simulink model "version4_dq"  (R2023b)
settings: Solver=VariableStepAuto  StartTime=0.0  StopTime=40  FixedStep=Ts_power  MaxStep=Ts_power  RelTol=1e-3
undefined symbols (not defined in the file): C_dc, c_dc, c_drt, c_f, C_hv_km, C_p_opt, Cagg, Cbase1v, H_gen, H_vsm, H_WTR, Ibase_hv, Ibase_lv, Ibase_mv, k_d_vsm, k_drt, k_p_p_vsm, k_p_q_vsm, K_pitch, ki_q, Kp_cc, kp_dc, kpu, L_comp, L_d, l_f, l_grid, L_hv_km, L_q, l_t_ehvhv, l_t_hvmv, l_t_mvlv, Lagg, lambda_opt, Lbase1v, length_export, omega_nom, omega_WTR_min, omega_WTR_n, omega_WTR_sl, phase_shift_test_state, phase_shifts, pie_export, pitch_max, pitch_min, Pitchanglevector, Powercoefficient, psi_pm, R_a, r_f, r_grid, R_hv_km, r_t_ehvhv, r_t_hvmv, r_t_mvlv, R_WTR, Ragg, rate_max, rate_min, rocof_slope ... (+22)
libraries: slpidlib x6, simulink x2, spsFirstOrderFilterLib x1, spsSampleandHoldLib x1
(part 1 of 3)
settings Model: SimulationMode=accelerator  Creator=Martin Pedersen  LastModifiedBy=Martin Pedersen
settings SolverCC: DecoupledContinuousIntegration=on
settings DataIOCC: InitialState=xu134_wWT  SaveFinalState=on  SaveFormat=Structure  SaveOutput=off  SignalLogging=off  DSMLogging=off  ReturnWorkspaceOutputs=off

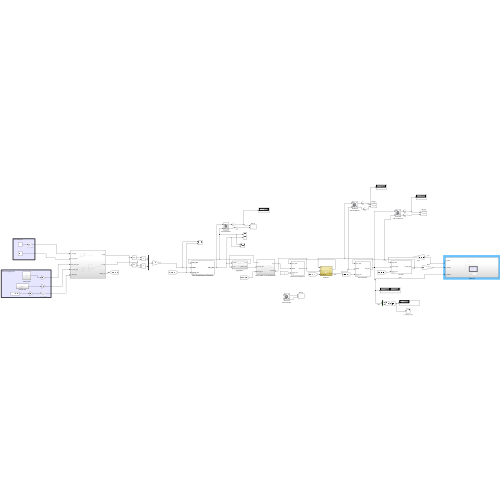
[thumbnail: Simulink's stored preview of the top-level diagram]
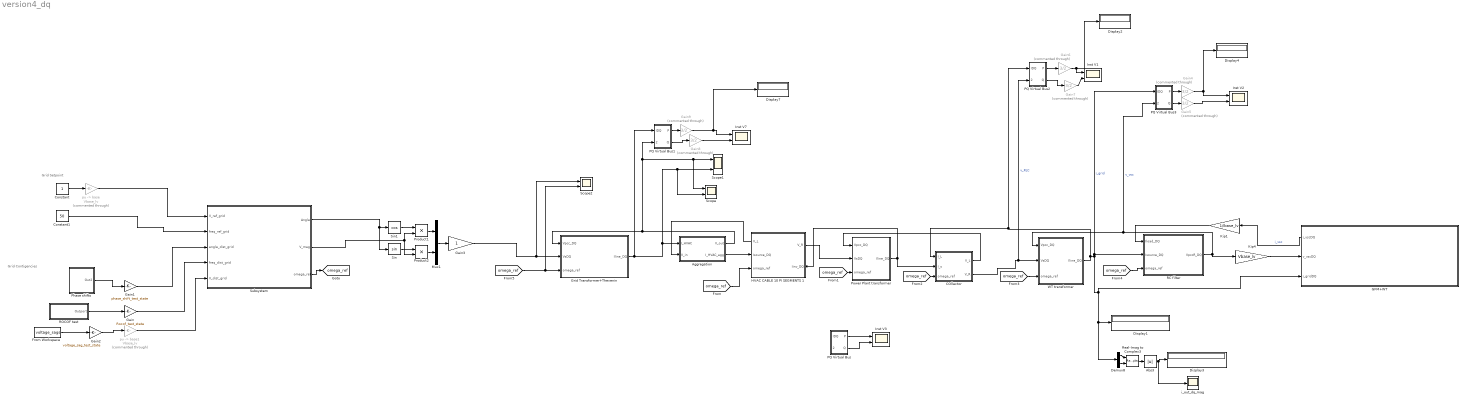
== system version4_dq ==
  note: Grid Contigencies
  note: Grid Setpoint
  Abs3 : Abs
  Aggregation : Subsystem
  COllector : Subsystem
  Constant : Constant
  Constant1 : Constant  Value=50
  Demux8 : Demux  Outputs=[vect vect]
  Display{1..4,7} (5 alike) : Display
  From Workspace : FromWorkspace  VariableName=voltage_sags
  GFM+WT : Subsystem
      settings: PortSchema="{\"entries\":[{\"content\":{\"sides\":[{\"content\":{\"connectorIds\":[\"Out1\",\"In1\",\"In2\"]},\"type\":\"ConnectorPlacement.EquallySpacedRectSide\",\"uuid\":\"bf5f9628-3d85-42f3-b508-ee12217f2900\"},{\"content\":{\"side\":\"RIGHT\"},\"type\":\"ConnectorPlacement.EquallySpacedRectSide\",\"uuid\":\"cb708a52-84f5-4fa8-a61c-6d72c4b87b86\"},{\"content\":{\"side\":\"TOP\"},\"type\":\"ConnectorPlacement.EquallySpacedRectSide\",\"uuid\":\"4c99ef60-a9c3-4166-9091-666343de6d32\"}]},\"type\":\"ConnectorPlacement.EquallySpacedConnector\",\"uuid\":\"b70419d4-69f8-4ca8-a89d-556a2a8c13e9\"}],\"packageUris\":[\"http://schema.mathworks.com/mf0/Connector/R2020b\"],\"version\":\"1.0\"}"
  Gain : Gain  Gain=Rocof_test_state
  Gain1 : Gain  Gain=phase_shift_test_state
  Gain2 : Gain  Gain=voltage_sag_test_state
  Gain3 : Gain  SaturateOnIntegerOverflow=on  OutDataTypeStr=Inherit: Same as input  ParamDataTypeStr=Inherit: Same as input
  Gain{4..9} (6 alike) : Gain  Commented=through  Gain=3/2
  Grid Transformer+Thevenin : Subsystem  mask{Rsource=r_grid+r_t_ehvhv, Lsource=(l_grid+l_t_ehvhv)/omega_nom}
      mask prompts: Rsource "Line resistance"; Lsource "line inductance"
      mask help:
      | RLV_NET is an 3 phase series RL with no virtual resistance termination,
      | 2 voltages as inputs and 1 current output
      mask init:
      | inv_Lsource=1/Lsource;
      mask TypeOptions Rsource: 2/Gain | 3/Gain
      mask TypeOptions Lsource: 7/Gain
  HVAC CABLE 10 PI SEGMENTS 1 : Subsystem
      settings: PortSchema="{\"entries\":[{\"content\":{\"sides\":[{\"content\":{\"connectorIds\":[\"Out2\",\"In1\",\"In2\"]},\"type\":\"ConnectorPlacement.EquallySpacedRectSide\",\"uuid\":\"364e0a5e-18fb-4479-9cea-0c32c2a31756\"},{\"content\":{\"connectorIds\":[\"Out1\",\"In3\"],\"side\":\"RIGHT\"},\"type\":\"ConnectorPlacement.EquallySpacedRectSide\",\"uuid\":\"1b6ff004-fcad-4add-afdc-525ba11bb75d\"},{\"content\":{\"side\":\"TOP\"},\"type\":\"ConnectorPlacement.EquallySpacedRectSide\",\"uuid\":\"fcc13093-d95c-447e-b2c0-1261755b0002\"}]},\"type\":\"ConnectorPlacement.EquallySpacedConnector\",\"uuid\":\"424862c2-d061-479a-b3c0-8c92e3670b7a\"}],\"packageUris\":[\"http://schema.mathworks.com/mf0/Connector/R2020b\"],\"version\":\"1.0\"}"
  Inst V{1..3,7} (4 alike) : Scope  NumInputPorts=2
  Kip1 : Gain  Gain=1/Ibase_lv
  Kip4 : Gain  Gain=Vbase_lv
  Mux1 : Mux  Inputs=2
  PQ Virtual Bus : Subsystem
  PQ Virtual Bus1 : Subsystem
  PQ Virtual Bus2 : Subsystem
  PQ Virtual Bus3 : Subsystem
  Phase shifts : Subsystem
  Power Plant transformer : Subsystem  mask{Rsource=r_t_hvmv, Lsource=l_t_hvmv/omega_nom}
      mask prompts: Rsource "Line resistance"; Lsource "line inductance"
      mask help:
      | RLV_NET is an 3 phase series RL with no virtual resistance termination,
      | 2 voltages as inputs and 1 current output
      mask init:
      | inv_Lsource=1/Lsource;
      mask TypeOptions Rsource: 2/Gain | 3/Gain
      mask TypeOptions Lsource: 7/Gain
  Product1 : Product
  Product2 : Product
  RC filter : Subsystem  mask{Csource=c_f/omega_nom, Rd=0, VD0=1, VQ0=0}
      mask prompts: Csource "Net Capacitance"; Rd "Rdamp"
      mask help:
      | PI network, capacitance to enter is total.
      | Left and right current as input. Left and right voltage as output
      mask init:
      | inv_Csource=1/Csource;
      mask TypeOptions Csource: 8/Gain
      mask TypeOptions Rd: 1/Gain | 2/Gain
      mask TypeOptions VD0: VcpdR_int/InitialCondition
      mask TypeOptions VQ0: VcpqR_int/InitialCondition
  ROCOF test : Subsystem
  Real-Imag to Complex3 : RealImagToComplex
  Scope : Scope  NumInputPorts=2
  Scope1 : Scope  NumInputPorts=2
  Scope2 : Scope  NumInputPorts=2
  Sin : Trigonometry
  Sin1 : Trigonometry  Operator=cos
  Subsystem : Subsystem
  "WT transformer " : Subsystem  mask{Rsource=r_t_mvlv, Lsource=l_t_mvlv/omega_nom}
      mask prompts: Rsource "Line resistance"; Lsource "line inductance"
      mask help:
      | RLV_NET is an 3 phase series RL with no virtual resistance termination,
      | 2 voltages as inputs and 1 current output
      mask init:
      | inv_Lsource=1/Lsource;
      mask TypeOptions Rsource: 2/Gain | 3/Gain
      mask TypeOptions Lsource: 7/Gain
  i_out_dq_mag : Scope
  "pu -> base" : Gain  Commented=through  Gain=Vbase_lv
  "pu -> base1" : Gain  Commented=through  Gain=Vbase_lv
  tag scope: omega_ref=global
  wires:
  Sin/1 -> Product2/1
  Product2/1 -> Mux1/2
  Phase shifts/1(Out2) -> Gain1/1
  Product1/1 -> Mux1/1
  Gain2/1 -> "pu -> base1"/1
  Gain1/1 -> Subsystem/3(angle_dist_grid)
  "pu -> base1"/1 -> Subsystem/5(V_dist_grid)
  ROCOF test/1(Outport) -> Gain/1
  Subsystem/3(omega_ref) -> [omega_ref]
  Subsystem/1(Angle) -> Sin/1, Sin1/1
  Constant/1 -> "pu -> base"/1
  Subsystem/2(V_mag) -> Product2/2, Product1/2
  "pu -> base"/1 -> Subsystem/1(V_ref_grid)
  Mux1/1 -> Gain3/1
  Constant1/1 -> Subsystem/2(freq_ref_grid)
  Sin1/1 -> Product1/1
  Gain/1 -> Subsystem/4(freq_dist_grid)
  From Workspace/1 -> Gain2/1
  Gain3/1 -> Scope2/1, Grid Transformer+Thevenin/2("VsDQ ")
  [omega_ref] -> RC filter/3(omega_ref)
  [omega_ref] -> HVAC CABLE 10 PI SEGMENTS 1/2(omega_ref)
  [omega_ref] -> Power Plant transformer/3(omega_ref)
  PQ Virtual Bus2/2(Q) -> Gain7/1
  PQ Virtual Bus1/1(P) -> Gain9/1
  Gain8/1 -> Inst V7/2
  Gain9/1 -> Display7/1, Inst V7/1
  Real-Imag to Complex3/1 -> Abs3/1
  Gain7/1 -> Inst V1/2
  [omega_ref] -> Scope2/2, Grid Transformer+Thevenin/3(omega_ref)
  COllector/2(V_R) -> PQ Virtual Bus2/2(VDQ), "WT transformer "/2("VsDQ ")  "v_RLC"
  Gain6/1 -> Inst V1/1, Display2/1
  PQ Virtual Bus3/2(Q) -> Gain5/1
  Aggregation/2(I_HVAC_agg) -> HVAC CABLE 10 PI SEGMENTS 1/1("Isource_DQ ")
  PQ Virtual Bus/2(Q) -> Inst V3/2
  PQ Virtual Bus2/1(P) -> Gain6/1
  PQ Virtual Bus3/1(P) -> Gain4/1
  Gain5/1 -> Inst V2/2
  RC filter/1(VpccR_DQ) -> "WT transformer "/1(Vpcc_DQ), PQ Virtual Bus3/2(VDQ), Kip4/1  "v_vsc"
  [omega_ref] -> COllector/3(omega_ref)
  Demux8/2 -> Real-Imag to Complex3/2
  [omega_ref] -> "WT transformer "/3(omega_ref)
  GFM+WT/1(i_vscDQ) -> Kip1/1  "i_vsc"
  HVAC CABLE 10 PI SEGMENTS 1/1(V_R) -> Power Plant transformer/2("VsDQ ")
  Abs3/1 -> i_out_dq_mag/1, Display3/1
  PQ Virtual Bus/1(P) -> Inst V3/1
  Aggregation/1(V_out) -> PQ Virtual Bus1/2(VDQ), Scope/1, Scope1/1, Grid Transformer+Thevenin/1(Vpcc_DQ)
  PQ Virtual Bus1/2(Q) -> Gain8/1
  HVAC CABLE 10 PI SEGMENTS 1/2(V_L) -> Aggregation/2(V_in)
  Demux8/1 -> Real-Imag to Complex3/1
  Gain4/1 -> Display4/1, Inst V2/1
  COllector/1(V_L) -> Power Plant transformer/1(Vpcc_DQ)
  Power Plant transformer/1(Iline_DQ) -> COllector/2(I_s), HVAC CABLE 10 PI SEGMENTS 1/3(Iinv_DQ)
  "WT transformer "/1(Iline_DQ) -> PQ Virtual Bus2/1(IDQ), COllector/1(I_L), GFM+WT/2(i_gridDQ), Demux8/1, Display1/1, RC filter/2("Isource_DQ "), PQ Virtual Bus3/1(IDQ)  "i_grid"
  Grid Transformer+Thevenin/1(Iline_DQ) -> Aggregation/1(I_HVAC), Scope/2, Scope1/2, PQ Virtual Bus1/1(IDQ)
  Kip4/1 -> GFM+WT/1(v_vscDQ)
  Kip1/1 -> RC filter/1(Iload_DQ)

== system version4_dq/Aggregation ==
  I_HVAC : Inport
  V_in : Inport  Port=2
  Demux1 : Demux  Outputs=[vect vect]
  Demux2 : Demux  Outputs=2
  Gain2 : Gain  Gain=1/(1*vect)
  Gain3 : Gain  Gain=ones(vect,1)
  Gain4 : Gain  Gain=ones(vect,1)
  Mux2 : Mux  Inputs=2
  Mux3 : Mux  Inputs=2
  Sum of Elements : Sum  Inputs=+
  Sum of Elements1 : Sum  Inputs=+
  V_out : Outport
  I_HVAC_agg : Outport  Port=2
  wires:
  Mux3/1 -> Gain2/1
  Gain3/1 -> Mux2/1
  Demux2/1 -> Gain3/1
  Sum of Elements1/1 -> Mux3/2
  Gain4/1 -> Mux2/2
  Demux2/2 -> Gain4/1
  Sum of Elements/1 -> Mux3/1
  Gain2/1 -> I_HVAC_agg/1
  V_in/1 -> Demux2/1
  Mux2/1 -> V_out/1
  I_HVAC/1 -> Demux1/1
  Demux1/1 -> Sum of Elements/1
  Demux1/2 -> Sum of Elements1/1

== system version4_dq/COllector ==
  I_L : Inport
  I_s : Inport  Port=2
  omega_ref : Inport  Port=3
  Gain2 : Gain  Gain=1/Vbase_mv
  Gain3 : Gain  Gain=1/Vbase_mv
  Gain4 : Gain  Gain=Ibase_mv
  Gain5 : Gain  Gain=Ibase_mv
  Scope : Scope  NumInputPorts=2
  collector : Subsystem  mask{Rsource=Ragg, Csource=Cagg, Lsource=Lagg}
      mask prompts: Rsource "Series R"; Csource "Net Capacitance"; Lsource "Net Inductance"
      mask help:
      | PI network, capacitance to enter is total.
      | Left and right current as input. Left and right voltage as output
      mask init:
      | inv_Csource=2/Csource;
      | inv_Lsource=1/Lsource;
      mask TypeOptions Rsource: 2/Gain | 3/Gain
      mask TypeOptions Csource: 8/Gain
      mask TypeOptions Lsource: 7/Gain
  V_L : Outport
  V_R : Outport  Port=2
  wires:
  Gain4/1 -> collector/1(Iload_DQ)
  collector/1(VpccR_DQ) -> Gain2/1
  Gain2/1 -> V_R/1
  collector/2(VpccL_DQ) -> Gain3/1
  I_s/1 -> Gain5/1
  Gain3/1 -> Scope/1, V_L/1
  Gain5/1 -> collector/2("Isource_DQ ")
  I_L/1 -> Scope/2, Gain4/1
  omega_ref/1 -> collector/3(omega_ref)

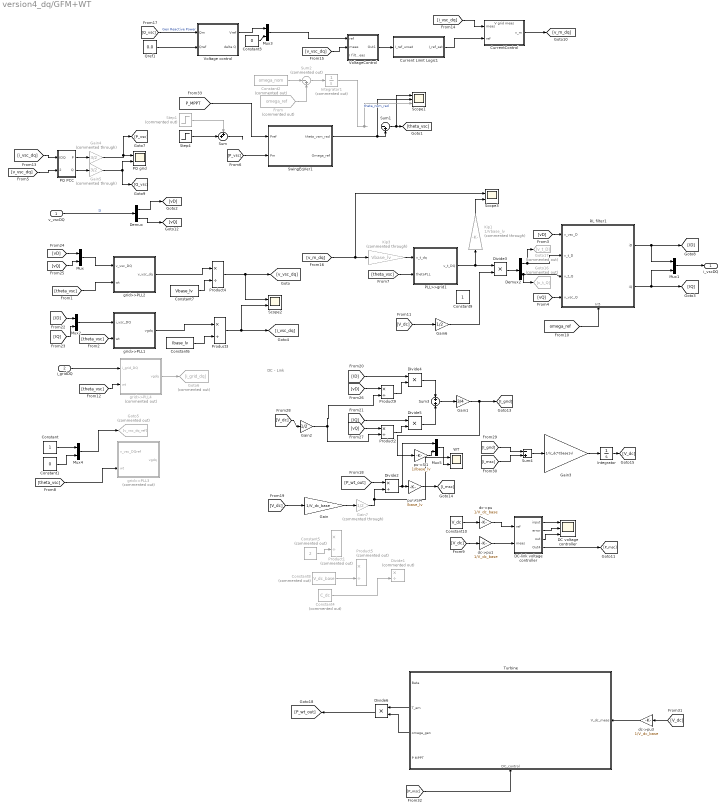
== system version4_dq/GFM+WT ==
  note: DC - Link
  v_vscDQ : Inport
  i_gridDQ : Inport  Port=2
  Constant : Constant
  Constant1 : Constant  Value=0
  Constant10 : Constant  Value=V_dc
  Constant2 : Constant  Commented=on  Value=omega_nom
  Constant3 : Constant  Value=0
  Constant4 : Constant  Commented=on  Value=C_dc  SampleTime=Ts_power
  Constant5 : Constant  Commented=on  Value=2  SampleTime=Ts_power
  Constant6 : Constant  Value=Ibase_lv
  Constant7 : Constant  Value=Vbase_lv
  Constant8 : Constant  Commented=on  Value=V_dc_base  SampleTime=Ts_power
  Constant9 : Constant
  Current Limit Logic1 : Subsystem
  CurrentControl : Subsystem
      settings: PortSchema="{\"entries\":[{\"content\":{\"sides\":[{\"content\":{\"connectorIds\":[\"In1\",\"In2\"]},\"type\":\"ConnectorPlacement.EquallySpacedRectSide\",\"uuid\":\"219db9ea-637c-42c0-b87e-0a8373949a2f\"},{\"content\":{\"connectorIds\":[\"Out1\"],\"side\":\"RIGHT\"},\"type\":\"ConnectorPlacement.EquallySpacedRectSide\",\"uuid\":\"817edf77-a627-4761-8536-4c41ccdce557\"},{\"content\":{\"side\":\"TOP\"},\"type\":\"ConnectorPlacement.EquallySpacedRectSide\",\"uuid\":\"b4d64eff-9104-48e3-a4e2-ec81b224adc3\"},{\"content\":{\"connectorIds\":[\"In3\"],\"side\":\"BOTTOM\"},\"type\":\"ConnectorPlacement.EquallySpacedRectSide\",\"uuid\":\"8db682a6-86bb-4d51-9cc3-8f643a502240\"}]},\"type\":\"ConnectorPlacement.EquallySpacedConnector\",\"uuid\":\"cfbf309f-cee6-401c-8c28-748b4359d9c9\"}],\"packageUris\":[\"http://schema.mathworks.com/mf0/Connector/R2020b\"],\"version\":\"1.0\"}"
  DC voltage controller : Scope  NumInputPorts=3
  DC-link voltage controller : Subsystem
  Demux : Demux  Outputs=2
  Demux2 : Demux  Outputs=2
  Divide1 : Product  Commented=on  Inputs=*/
  Divide2 : Product  Inputs=*/
  Divide{3..6} (4 alike) : Product  Inputs=**
  From : From  Commented=on  GotoTag=omega_ref  TagVisibility=global
  Gain : Gain  Gain=1/V_dc_base
  Gain1 : Gain  Gain=3/4
  Gain2 : Gain  Gain=1/2
  Gain3 : Gain  Gain=1/(c_dc*Cbase1v)
  Gain4 : Gain  Commented=through  Gain=3/2
  Gain5 : Gain  Commented=through  Gain=3/2
  Gain6 : Gain  Gain=1/2
  Gain7 : Gain  Commented=through  Gain=1/2
  Goto16 : Goto  Commented=on  GotoTag=v_t_Q
  Goto17 : Goto  Commented=on  GotoTag=v_t_D
  Goto5 : Goto  Commented=on  GotoTag=v_vsc_dq_ref
  Goto6 : Goto  Commented=on  GotoTag=i_grid_dq
  Integrator : Integrator  InitialCondition=V_dc  ContinuousStateAttributes='Delta_v_dc'
  Integrator1 : Integrator  Commented=on  WrappedStateUpperValue=2*pi  WrappedStateLowerValue=0
  Kip1 : Gain  Commented=through  Gain=1/Vbase_lv
  Kip3 : Gain  Commented=through  Gain=Vbase_lv
  Mux{,1,3,5} (4 alike) : Mux  Inputs=2
  Mux2 : Mux  Inputs=[vect vect]
  Mux4 : Mux  Inputs=[vect vect]
  PLL>>grid1 : Subsystem  AncestorBlock=powerlib_meascontrol/Transformations/Alpha-Beta-Zero to dq0/Subsystem - pi//2 delay
  PQ PCC : Subsystem
  PQ grid : Scope  NumInputPorts=2
  Product1 : Product  Commented=on  Inputs=*/
  Product{2..4,9} (4 alike) : Product  Inputs=*/
  Product5 : Product  Commented=on  Inputs=*/
  Qref1 : Constant  Value=0.0
  RL filter1 : Subsystem
      settings: PortSchema="{\"entries\":[{\"content\":{\"sides\":[{\"content\":{\"connectorIds\":[\"In1\",\"In2\",\"In3\",\"In4\"]},\"type\":\"ConnectorPlacement.EquallySpacedRectSide\",\"uuid\":\"57ad71d1-5664-4b35-a20c-d71f7e1cdc47\"},{\"content\":{\"connectorIds\":[\"Out1\",\"Out2\"],\"side\":\"RIGHT\"},\"type\":\"ConnectorPlacement.EquallySpacedRectSide\",\"uuid\":\"8101605d-eedb-4c26-847d-0cc0ce629d60\"},{\"content\":{\"side\":\"TOP\"},\"type\":\"ConnectorPlacement.EquallySpacedRectSide\",\"uuid\":\"2627b00b-24a5-469a-be2d-9c3c8a1d2080\"},{\"content\":{\"connectorIds\":[\"In5\"],\"side\":\"BOTTOM\"},\"type\":\"ConnectorPlacement.EquallySpacedRectSide\",\"uuid\":\"fe553db7-7727-4a02-b1e7-5aedfb7840ee\"}]},\"type\":\"ConnectorPlacement.EquallySpacedConnector\",\"uuid\":\"f40200c8-ad5b-428c-8a4e-7641595b86c4\"}],\"packageUris\":[\"http://schema.mathworks.com/mf0/Connector/R2020b\"],\"version\":\"1.0\"}"
  Scope1 : Scope  NumInputPorts=3
  Scope2 : Scope  NumInputPorts=2
  Scope3 : Scope  NumInputPorts=2
  Step1 : Step  Commented=on  Time=3.5  After=0.2  SampleTime=0
  Step4 : Step  After=0.58  SampleTime=0
  Sum : Sum  Inputs=++|
  Sum1 : Sum  Inputs=|-+
  Sum2 : Sum  Commented=on  Inputs=|-+
  Sum3 : Sum  Inputs=+|+
  Sum4 : Sum  Inputs=-+
  SwingEqVer1 : Subsystem
  Turbine : Subsystem
      settings: PortSchema="{\"entries\":[{\"content\":{\"sides\":[{\"content\":{\"connectorIds\":[\"In1\"]},\"type\":\"ConnectorPlacement.EquallySpacedRectSide\",\"uuid\":\"21e34078-e55f-4d30-b877-fe893009bf50\"},{\"content\":{\"connectorIds\":[\"Out1\",\"Out2\",\"Out3\",\"Out4\"],\"side\":\"RIGHT\"},\"type\":\"ConnectorPlacement.EquallySpacedRectSide\",\"uuid\":\"7fcce3d7-4700-4aed-9466-c9df21636c23\"},{\"content\":{\"side\":\"TOP\"},\"type\":\"ConnectorPlacement.EquallySpacedRectSide\",\"uuid\":\"1e7dcbfc-6914-4635-b5b6-37bd72b5c977\"},{\"content\":{\"connectorIds\":[\"In2\"],\"side\":\"BOTTOM\"},\"type\":\"ConnectorPlacement.EquallySpacedRectSide\",\"uuid\":\"4cd2ac35-fe5e-4d2f-8870-f4b31c475178\"}]},\"type\":\"ConnectorPlacement.EquallySpacedConnector\",\"uuid\":\"0de0e372-1be9-4afb-8b34-f97f900b0306\"}],\"packageUris\":[\"http://schema.mathworks.com/mf0/Connector/R2020b\"],\"version\":\"1.0\"}"
  Voltage control : Subsystem
  VoltageControl : Subsystem
  WT : Scope  NumInputPorts=2
  dc->pu : Gain  Gain=1/V_dc_base
  dc->pu1 : Gain  Gain=1/V_dc_base
  dc->pu3 : Gain  Gain=1/V_dc_base
  grid>>PLL1 : Subsystem  AncestorBlock=powerlib_meascontrol/Transformations/dq0 to Alpha-Beta-Zero/Subsystem1
  grid>>PLL2 : Subsystem  AncestorBlock=powerlib_meascontrol/Transformations/dq0 to Alpha-Beta-Zero/Subsystem1
  grid>>PLL3 : Subsystem  Commented=on  AncestorBlock=powerlib_meascontrol/Transformations/dq0 to Alpha-Beta-Zero/Subsystem1
  grid>>PLL4 : Subsystem  Commented=on  AncestorBlock=powerlib_meascontrol/Transformations/dq0 to Alpha-Beta-Zero/Subsystem1
  pu->SI1 : Gain  Gain=1/Ibase_lv
  pu->SI4 : Gain  Gain=Ibase_lv
  i_vscDQ : Outport
  wires:
  Demux/2 -> [vQ]
  Demux/1 -> [vD]
  [vQ] -> Mux/2
  [vD] -> Mux/1
  Mux1/1 -> i_vscDQ/1
  [ID] -> Mux2/1
  [IQ] -> Mux2/2
  Mux2/1 -> grid>>PLL1/1(i_vsc_DQ)
  From/1 -> Sum2/2
  SwingEqVer1/1(theta_vsm_rad) -> Sum1/2, Scope1/2
  Sum1/1 -> Scope1/1, [theta_vsc]
  [theta_vsc] -> grid>>PLL2/2(wt)
  [theta_vsc] -> grid>>PLL1/2(wt)
  PQ PCC/1(P) -> Gain4/1
  RL filter1/1(iD) -> Mux1/1, [ID]
  RL filter1/2(iQ) -> Mux1/2, [IQ]
  Mux/1 -> grid>>PLL2/1(v_vsc_DQ)
  [vD] -> RL filter1/1(v_vsc_D)
  [vQ] -> RL filter1/4(v_vsc_Q)
  grid>>PLL2/1(v_vsc_dq) -> Product4/1
  [i_vsc_dq] -> PQ PCC/1(IDQ)
  grid>>PLL1/1(vgdq) -> Product3/1
  Step1/1 -> Sum/1
  Step4/1 -> Sum/2
  Kip3/1 -> PLL>>grid1/1(v_t_dq)
  Demux2/1 -> Goto17/1, RL filter1/2(v_t_D)
  Constant/1 -> Mux4/1
  Constant1/1 -> Mux4/2
  Mux4/1 -> Goto5/1
  [v_m_dq] -> Scope3/1, Kip3/1
  [omega_ref] -> RL filter1/5(In5)
  i_gridDQ/1 -> grid>>PLL4/1(i_grid_DQ)
  [theta_vsc] -> grid>>PLL4/2(wt)
  grid>>PLL4/1(vgdq) -> Goto6/1
  Constant2/1 -> Sum2/1
  Sum2/1 -> Integrator1/1
  [v_vsc_dq] -> PQ PCC/2(VDQ)
  v_vscDQ/1 -> Demux/1  "SI"
  Product4/1 -> [v_vsc_dq], Scope2/1
  PLL>>grid1/1(v_t_DQ) -> Kip1/1, Divide3/1
  Product3/1 -> Scope2/2, [i_vsc_dq]
  PQ PCC/2(Q) -> Gain5/1
  [theta_vsc] -> grid>>PLL3/2(wt)
  [theta_vsc] -> PLL>>grid1/2(thetaPLL)
  [P_vsc] -> SwingEqVer1/2(Pm)
  VoltageControl/1(Out1) -> Current Limit Logic1/1(I_ref_unsat)
  [i_vsc_dq] -> CurrentControl/2(meas)
  [v_vsc_dq] -> VoltageControl/2(meas)
  Mux3/1 -> VoltageControl/1(ref)
  CurrentControl/1(v_m) -> [v_m_dq]
  Qref1/1 -> Voltage control/2(Qref)
  [Q_vsc] -> Voltage control/1(Qm)  "Gen Reactive Power"
  Voltage control/1(Vref) -> Mux3/1
  Constant3/1 -> Mux3/2
  DC-link voltage controller/4(Out4) -> [P_msc]
  DC-link voltage controller/3(out) -> DC voltage controller/3
  DC-link voltage controller/1(input) -> DC voltage controller/1
  dc->pu1/1 -> DC-link voltage controller/2(meas)
  Constant10/1 -> dc->pu/1
  DC-link voltage controller/2(error) -> DC voltage controller/2
  [V_dc] -> dc->pu1/1
  dc->pu/1 -> DC-link voltage controller/1(ref)
  Gain/1 -> Gain7/1
  [V_dc] -> Gain/1
  [P_wt_out] -> Divide2/1
  Divide2/1 -> Mux5/1, pu->SI4/1
  [V_dc] -> Gain6/1
  Gain3/1 -> Integrator/1
  [vD] -> Product9/1
  [vQ] -> Product2/1
  Gain2/1 -> Product9/2, Product2/2
  [V_dc] -> Gain2/1
  [ID] -> Divide4/1
  Product9/1 -> Divide4/2
  [IQ] -> Divide5/1
  Product2/1 -> Divide5/2
  Divide4/1 -> Sum3/1
  Divide5/1 -> Sum3/2
  Sum3/1 -> Gain1/1
  pu->SI4/1 -> [I_msc]
  Sum4/1 -> Gain3/1
  [I_msc] -> Sum4/2
  [I_grid] -> Sum4/1
  Integrator/1 -> [V_dc]
  Divide3/1 -> Demux2/1
  Demux2/2 -> Goto16/1, RL filter1/3(v_t_Q)
  Constant6/1 -> Product3/2
  Constant7/1 -> Product4/2
  Constant8/1 -> Product5/2
  Constant5/1 -> Product1/2
  Constant4/1 -> Divide1/2
  dc->pu3/1 -> Turbine/1(V_dc_meas)
  [V_dc] -> dc->pu3/1
  [P_msc] -> Turbine/2(DC_control)
  Turbine/3(omega_gen) -> Divide6/2
  ? -> ?
  Turbine/2(T_em) -> Divide6/1
  pu->SI1/1 -> Mux5/2
  Mux5/1 -> WT/2
  Gain1/1 -> pu->SI1/1, [I_grid]
  Kip1/1 -> Scope3/2
  Divide6/1 -> [P_wt_out]
  Gain4/1 -> [P_vsc], PQ grid/1
  Gain5/1 -> PQ grid/2, [Q_vsc]
  [P_MPPT] -> SwingEqVer1/1(Pref)
  Sum/1 -> ?
  Integrator1/1 -> Scope1/3  "theta_nom_rad"
  Current Limit Logic1/1(I_ref_sat) -> CurrentControl/1(ref)
  Gain6/1 -> Divide3/2
  Gain7/1 -> WT/1, Divide2/2

== system version4_dq/Grid Transformer+Thevenin ==
  note: Network
  note: VIRTUAL RESITANCE
  Vpcc_DQ : Inport
  "VsDQ " : Inport  Port=2
  omega_ref : Inport  Port=3
  1 : Gain  Gain=inv_Lsource
  2 : Gain  Gain=Rsource
  3 : Gain  Gain=Rsource
  4 : Gain  Gain=inv_Lsource
  7 : Gain  Gain=Lsource
  Demux1 : Demux  Outputs=2
  Demux2 : Demux  Outputs=2
  Id : Scope
  Iline_D_int : Integrator  UpperSaturationLimit=50  LowerSaturationLimit=-1000
  Iline_Q_int : Integrator  UpperSaturationLimit=50  LowerSaturationLimit=-1000
  Iq : Scope
  Mux1 : Mux  Inputs=2
  Mux4 : Mux  Inputs=2
  Product1 : Product
  Product2 : Product
  Sum1 : Sum  Inputs=|+---
  Sum8 : Sum  Inputs=|+-+-
  Iline_DQ : Outport  VectorParamsAs1DForOutWhenUnconnected=off
  wires:
  7/1 -> [wL]
  omega_ref/1 -> 7/1
  [Vpcc_Q] -> Sum1/1
  [Vpcc_D] -> Sum8/1
  Demux2/1 -> Mux4/1, [Vpcc_D]
  Demux2/2 -> Mux4/2, [Vpcc_Q]
  Sum1/1 -> 4/1
  1/1 -> Iline_D_int/1
  Iline_D_int/1 -> Product1/2, Id/1, 2/1, Mux1/1
  Iline_Q_int/1 -> Mux1/2, Iq/1, Product2/2, 3/1
  Sum8/1 -> 1/1
  2/1 -> Sum8/4
  Product2/1 -> Sum8/3
  3/1 -> Sum1/4
  4/1 -> Iline_Q_int/1
  Product1/1 -> Sum1/3
  [wL] -> Product1/1, Product2/1
  Demux1/1 -> Sum8/2
  Demux1/2 -> Sum1/2
  "VsDQ "/1 -> Demux1/1
  Vpcc_DQ/1 -> Demux2/1
  Mux1/1 -> Iline_DQ/1

== system version4_dq/HVAC CABLE 10 PI SEGMENTS 1 ==
  "Isource_DQ " : Inport
  omega_ref : Inport  Port=2
  Iinv_DQ : Inport  Port=3
  Gain1 : Gain  Gain=1/Vbase_hv
  Gain2 : Gain  Gain=1/Vbase_hv
  Gain4 : Gain  Gain=Ibase_hv
  Gain5 : Gain  Gain=Ibase_hv
  RC sys1 : Subsystem  mask{Csource=C_hv_km*length_export/pie_export/2, Rd=0.00001, VD0=1, VQ0=0}
      mask prompts: Csource "Net Capacitance"; Rd "Rdamp"
      mask help:
      | PI network, capacitance to enter is total.
      | Left and right current as input. Left and right voltage as output
      mask init:
      | inv_Csource=1/Csource;
      mask TypeOptions Csource: 8/Gain
      mask TypeOptions Rd: 1/Gain | 2/Gain
      mask TypeOptions VD0: VcpdR_int/InitialCondition
      mask TypeOptions VQ0: VcpqR_int/InitialCondition
  RLC_NET 11 : Subsystem  mask{Csource=C_hv_km*length_export/pie_export, Rsource=R_hv_km*length_export/pie_export, Lsource=L_hv_km*length_export/pie_export}
      mask prompts: Csource "line capacitance 1 side"; Rsource "Line resistance"; Lsource "line inductance"
      mask help:
      | RL with C terminations on right,
      | Left Voltage  and Right current input, Right voltage and left current output
      mask init:
      | inv_Csource=1/Csource;
      | inv_Lsource=1/Lsource;
      mask TypeOptions Csource: 8/Gain
      mask TypeOptions Rsource: 2/Gain | 3/Gain
      mask TypeOptions Lsource: 7/Gain
  RLC_NET 12 : Subsystem  mask{Csource=C_hv_km*length_export/pie_export, Rsource=R_hv_km*length_export/pie_export, Lsource=L_hv_km*length_export/pie_export}
      mask prompts: Csource "line capacitance 1 side"; Rsource "Line resistance"; Lsource "line inductance"
      mask help:
      | RL with C terminations on right,
      | Left Voltage  and Right current input, Right voltage and left current output
      mask init:
      | inv_Csource=1/Csource;
      | inv_Lsource=1/Lsource;
      mask TypeOptions Csource: 8/Gain
      mask TypeOptions Rsource: 2/Gain | 3/Gain
      mask TypeOptions Lsource: 7/Gain
  RLC_NET 13 : Subsystem  mask{Csource=C_hv_km*length_export/pie_export, Rsource=R_hv_km*length_export/pie_export, Lsource=L_hv_km*length_export/pie_export}
      mask prompts: Csource "line capacitance 1 side"; Rsource "Line resistance"; Lsource "line inductance"
      mask help:
      | RL with C terminations on right,
      | Left Voltage  and Right current input, Right voltage and left current output
      mask init:
      | inv_Csource=1/Csource;
      | inv_Lsource=1/Lsource;
      mask TypeOptions Csource: 8/Gain
      mask TypeOptions Rsource: 2/Gain | 3/Gain
      mask TypeOptions Lsource: 7/Gain
  RLC_NET 14 : Subsystem  mask{Csource=C_hv_km*length_export/pie_export, Rsource=R_hv_km*length_export/pie_export, Lsource=L_hv_km*length_export/pie_export}
      mask prompts: Csource "line capacitance 1 side"; Rsource "Line resistance"; Lsource "line inductance"
      mask help:
      | RL with C terminations on right,
      | Left Voltage  and Right current input, Right voltage and left current output
      mask init:
      | inv_Csource=1/Csource;
      | inv_Lsource=1/Lsource;
      mask TypeOptions Csource: 8/Gain
      mask TypeOptions Rsource: 2/Gain | 3/Gain
      mask TypeOptions Lsource: 7/Gain
  RLC_NET 15 : Subsystem  mask{Csource=C_hv_km*length_export/pie_export, Rsource=R_hv_km*length_export/pie_export, Lsource=L_hv_km*length_export/pie_export}
      mask prompts: Csource "line capacitance 1 side"; Rsource "Line resistance"; Lsource "line inductance"
      mask help:
      | RL with C terminations on right,
      | Left Voltage  and Right current input, Right voltage and left current output
      mask init:
      | inv_Csource=1/Csource;
      | inv_Lsource=1/Lsource;
      mask TypeOptions Csource: 8/Gain
      mask TypeOptions Rsource: 2/Gain | 3/Gain
      mask TypeOptions Lsource: 7/Gain
  RLC_NET 16 : Subsystem  mask{Csource=C_hv_km*length_export/pie_export, Rsource=R_hv_km*length_export/pie_export, Lsource=L_hv_km*length_export/pie_export}
      mask prompts: Csource "line capacitance 1 side"; Rsource "Line resistance"; Lsource "line inductance"
      mask help:
      | RL with C terminations on right,
      | Left Voltage  and Right current input, Right voltage and left current output
      mask init:
      | inv_Csource=1/Csource;
      | inv_Lsource=1/Lsource;
      mask TypeOptions Csource: 8/Gain
      mask TypeOptions Rsource: 2/Gain | 3/Gain
      mask TypeOptions Lsource: 7/Gain
  RLC_NET 17 : Subsystem  mask{Csource=C_hv_km*length_export/pie_export, Rsource=R_hv_km*length_export/pie_export, Lsource=L_hv_km*length_export/pie_export}
      mask prompts: Csource "line capacitance 1 side"; Rsource "Line resistance"; Lsource "line inductance"
      mask help:
      | RL with C terminations on right,
      | Left Voltage  and Right current input, Right voltage and left current output
      mask init:
      | inv_Csource=1/Csource;
      | inv_Lsource=1/Lsource;
      mask TypeOptions Csource: 8/Gain
      mask TypeOptions Rsource: 2/Gain | 3/Gain
      mask TypeOptions Lsource: 7/Gain
  RLC_NET 18 : Subsystem  mask{Csource=C_hv_km*length_export/pie_export, Rsource=R_hv_km*length_export/pie_export, Lsource=L_hv_km*length_export/pie_export}
      mask prompts: Csource "line capacitance 1 side"; Rsource "Line resistance"; Lsource "line inductance"
      mask help:
      | RL with C terminations on right,
      | Left Voltage  and Right current input, Right voltage and left current output
      mask init:
      | inv_Csource=1/Csource;
      | inv_Lsource=1/Lsource;
      mask TypeOptions Csource: 8/Gain
      mask TypeOptions Rsource: 2/Gain | 3/Gain
      mask TypeOptions Lsource: 7/Gain
  RLC_NET 19 : Subsystem  mask{Csource=C_hv_km*length_export/pie_export, Rsource=R_hv_km*length_export/pie_export, Lsource=L_hv_km*length_export/pie_export}
      mask prompts: Csource "line capacitance 1 side"; Rsource "Line resistance"; Lsource "line inductance"
      mask help:
      | RL with C terminations on right,
      | Left Voltage  and Right current input, Right voltage and left current output
      mask init:
      | inv_Csource=1/Csource;
      | inv_Lsource=1/Lsource;
      mask TypeOptions Csource: 8/Gain
      mask TypeOptions Rsource: 2/Gain | 3/Gain
      mask TypeOptions Lsource: 7/Gain
  RLC_NET 20 : Subsystem  mask{Csource=C_hv_km*length_export/pie_export/2, Rsource=R_hv_km*length_export/pie_export, Lsource=L_hv_km*length_export/pie_export}
      mask prompts: Csource "line capacitance 1 side"; Rsource "Line resistance"; Lsource "line inductance"
      mask help:
      | RL with C terminations on right,
      | Left Voltage  and Right current input, Right voltage and left current output
      mask init:
      | inv_Csource=1/Csource;
      | inv_Lsource=1/Lsource;
      mask TypeOptions Csource: 8/Gain
      mask TypeOptions Rsource: 2/Gain | 3/Gain
      mask TypeOptions Lsource: 7/Gain
  RLV_NET 1 : Subsystem  mask{Rsource=0, Lsource=L_comp}
      mask prompts: Rsource "Line resistance"; Lsource "line inductance"
      mask help:
      | RLV_NET is an 3 phase series RL with no virtual resistance termination,
      | 2 voltages as inputs and 1 current output
      mask init:
      | inv_Lsource=1/Lsource;
      mask TypeOptions Rsource: 2/Gain | 3/Gain
      mask TypeOptions Lsource: 7/Gain
  RLV_NET 2 : Subsystem  mask{Rsource=0, Lsource=L_comp}
      mask prompts: Rsource "Line resistance"; Lsource "line inductance"
      mask help:
      | RLV_NET is an 3 phase series RL with no virtual resistance termination,
      | 2 voltages as inputs and 1 current output
      mask init:
      | inv_Lsource=1/Lsource;
      mask TypeOptions Rsource: 2/Gain | 3/Gain
      mask TypeOptions Lsource: 7/Gain
  Sum2 : Sum  Inputs=++|
  Sum3 : Sum  Inputs=-+|
  V_R : Outport
  V_L : Outport  Port=2
  wires:
  RC sys1/1(VpccR_DQ) -> Gain1/1, RLV_NET 1/1(Vpcc_DQ), RLC_NET 11/2("VsDQ ")
  Gain1/1 -> V_L/1
  "Isource_DQ "/1 -> Gain4/1
  RLC_NET 11/1(Iline_DQ) -> RC sys1/1(Iload_DQ)
  Sum2/1 -> RC sys1/2("Isource_DQ ")
  Gain4/1 -> Sum2/2
  RLV_NET 1/1(Iline_DQ) -> Sum2/1
  omega_ref/1 -> [omega_ref]
  [omega_ref] -> RLC_NET 11/3(omega_ref)
  [omega_ref] -> RLC_NET 12/3(omega_ref)
  [omega_ref] -> RLC_NET 14/3(omega_ref)
  [omega_ref] -> RLC_NET 13/3(omega_ref)
  [omega_ref] -> RLC_NET 15/3(omega_ref)
  [omega_ref] -> RLC_NET 20/3(omega_ref)
  [omega_ref] -> RLC_NET 18/3(omega_ref)
  [omega_ref] -> RLC_NET 19/3(omega_ref)
  [omega_ref] -> RLC_NET 16/3(omega_ref)
  [omega_ref] -> RLC_NET 17/3(omega_ref)
  Iinv_DQ/1 -> Gain5/1
  Gain2/1 -> V_R/1
  RLC_NET 20/2(Vpcc_DQ) -> RLV_NET 2/1(Vpcc_DQ), Gain2/1
  Gain5/1 -> Sum3/2
  RLV_NET 2/1(Iline_DQ) -> Sum3/1
  [omega_ref] -> RLV_NET 2/2(omega_ref)
  RLC_NET 11/2(Vpcc_DQ) -> RLC_NET 12/2("VsDQ ")
  RLC_NET 12/1(Iline_DQ) -> RLC_NET 11/1(Iinv_DQ)
  RLC_NET 13/1(Iline_DQ) -> RLC_NET 12/1(Iinv_DQ)
  RLC_NET 12/2(Vpcc_DQ) -> RLC_NET 13/2("VsDQ ")
  RLC_NET 13/2(Vpcc_DQ) -> RLC_NET 14/2("VsDQ ")
  RLC_NET 14/1(Iline_DQ) -> RLC_NET 13/1(Iinv_DQ)
  RLC_NET 14/2(Vpcc_DQ) -> RLC_NET 15/2("VsDQ ")
  RLC_NET 15/1(Iline_DQ) -> RLC_NET 14/1(Iinv_DQ)
  RLC_NET 16/1(Iline_DQ) -> RLC_NET 15/1(Iinv_DQ)
  RLC_NET 17/1(Iline_DQ) -> RLC_NET 16/1(Iinv_DQ)
  RLC_NET 18/1(Iline_DQ) -> RLC_NET 17/1(Iinv_DQ)
  RLC_NET 16/2(Vpcc_DQ) -> RLC_NET 17/2("VsDQ ")
  RLC_NET 15/2(Vpcc_DQ) -> RLC_NET 16/2("VsDQ ")
  RLC_NET 19/1(Iline_DQ) -> RLC_NET 18/1(Iinv_DQ)
  RLC_NET 18/2(Vpcc_DQ) -> RLC_NET 19/2("VsDQ ")
  RLC_NET 17/2(Vpcc_DQ) -> RLC_NET 18/2("VsDQ ")
  RLC_NET 19/2(Vpcc_DQ) -> RLC_NET 20/2("VsDQ ")
  RLC_NET 20/1(Iline_DQ) -> RLC_NET 19/1(Iinv_DQ)
  Sum3/1 -> RLC_NET 20/1(Iinv_DQ)
  [omega_ref] -> RLV_NET 1/2(omega_ref), RC sys1/3(omega_ref)

== system version4_dq/PQ Virtual Bus ==
  note: PQ Virtual bus
  IDQ : Inport
  VDQ : Inport  Port=2
  Demux5 : Demux  Outputs=[vect vect]
  Demux6 : Demux  Outputs=[vect vect]
  Product{1,3..5} (4 alike) : Product  InputSameDT=on  SaturateOnIntegerOverflow=on  OutDataTypeStr=Inherit: Same as first input
  Sum : Sum  InputSameDT=on  SaturateOnIntegerOverflow=on  OutDataTypeStr=Inherit: Same as first input
  Sum1 : Sum  Inputs=+-  InputSameDT=on  SaturateOnIntegerOverflow=on  OutDataTypeStr=Inherit: Same as first input
  P : Outport
  Q : Outport  Port=2
  wires:
  Product3/1 -> Sum/1
  Demux5/2 -> Product4/2, Product5/2
  Product4/1 -> Sum/2
  Demux6/1 -> Product5/1, Product3/2
  Demux5/1 -> Product3/1, Product1/2
  Demux6/2 -> Product1/1, Product4/1
  Product1/1 -> Sum1/1
  Product5/1 -> Sum1/2
  Sum1/1 -> Q/1
  IDQ/1 -> Demux5/1
  VDQ/1 -> Demux6/1
  Sum/1 -> P/1

== system version4_dq/PQ Virtual Bus1 ==
  note: PQ Virtual bus
  IDQ : Inport
  VDQ : Inport  Port=2
  Demux5 : Demux  Outputs=[vect vect]
  Demux6 : Demux  Outputs=[vect vect]
  Product{1,3..5} (4 alike) : Product  InputSameDT=on  SaturateOnIntegerOverflow=on  OutDataTypeStr=Inherit: Same as first input
  Sum : Sum  InputSameDT=on  SaturateOnIntegerOverflow=on  OutDataTypeStr=Inherit: Same as first input
  Sum1 : Sum  Inputs=+-  InputSameDT=on  SaturateOnIntegerOverflow=on  OutDataTypeStr=Inherit: Same as first input
  P : Outport
  Q : Outport  Port=2
  wires:
  Product3/1 -> Sum/1
  Demux5/2 -> Product4/2, Product5/2
  Product4/1 -> Sum/2
  Demux6/1 -> Product5/1, Product3/2
  Demux5/1 -> Product3/1, Product1/2
  Demux6/2 -> Product1/1, Product4/1
  Product1/1 -> Sum1/1
  Product5/1 -> Sum1/2
  Sum1/1 -> Q/1
  IDQ/1 -> Demux5/1
  VDQ/1 -> Demux6/1
  Sum/1 -> P/1

== system version4_dq/PQ Virtual Bus2 ==
  note: PQ Virtual bus
  IDQ : Inport
  VDQ : Inport  Port=2
  Demux5 : Demux  Outputs=[vect vect]
  Demux6 : Demux  Outputs=[vect vect]
  Product{1,3..5} (4 alike) : Product  InputSameDT=on  SaturateOnIntegerOverflow=on  OutDataTypeStr=Inherit: Same as first input
  Sum : Sum  InputSameDT=on  SaturateOnIntegerOverflow=on  OutDataTypeStr=Inherit: Same as first input
  Sum1 : Sum  Inputs=+-  InputSameDT=on  SaturateOnIntegerOverflow=on  OutDataTypeStr=Inherit: Same as first input
  P : Outport
  Q : Outport  Port=2
  wires:
  Sum/1 -> P/1
  VDQ/1 -> Demux6/1
  IDQ/1 -> Demux5/1
  Sum1/1 -> Q/1
  Product5/1 -> Sum1/2
  Product1/1 -> Sum1/1
  Demux6/2 -> Product4/1, Product1/1
  Demux5/1 -> Product1/2, Product3/1
  Demux6/1 -> Product3/2, Product5/1
  Product4/1 -> Sum/2
  Demux5/2 -> Product5/2, Product4/2
  Product3/1 -> Sum/1

== system version4_dq/PQ Virtual Bus3 ==
  note: PQ Virtual bus
  IDQ : Inport
  VDQ : Inport  Port=2
  Demux5 : Demux  Outputs=[vect vect]
  Demux6 : Demux  Outputs=[vect vect]
  Product{1,3..5} (4 alike) : Product  InputSameDT=on  SaturateOnIntegerOverflow=on  OutDataTypeStr=Inherit: Same as first input
  Sum : Sum  InputSameDT=on  SaturateOnIntegerOverflow=on  OutDataTypeStr=Inherit: Same as first input
  Sum1 : Sum  Inputs=+-  InputSameDT=on  SaturateOnIntegerOverflow=on  OutDataTypeStr=Inherit: Same as first input
  P : Outport
  Q : Outport  Port=2
  wires:
  Product3/1 -> Sum/1
  Demux5/2 -> Product4/2, Product5/2
  Product4/1 -> Sum/2
  Demux6/1 -> Product5/1, Product3/2
  Demux5/1 -> Product3/1, Product1/2
  Demux6/2 -> Product1/1, Product4/1
  Product1/1 -> Sum1/1
  Product5/1 -> Sum1/2
  Sum1/1 -> Q/1
  IDQ/1 -> Demux5/1
  VDQ/1 -> Demux6/1
  Sum/1 -> P/1

== system version4_dq/Phase shifts ==
  Constant : Constant  Value=0
  From Workspace : FromWorkspace  Commented=on  VariableName=phase_shifts  OutputAfterFinalValue=Setting to zero
  Gain : Gain  Gain=-1
  Step : Step  Time=phase_shifts(1,1)  After=phase_shifts(1,2)  SampleTime=0
  Step1 : Step  Time=phase_shifts(2,1)  After=phase_shifts(2,2)  SampleTime=0
  Step2 : Step  Time=phase_shifts(3,1)  After=phase_shifts(3,2)  SampleTime=0
  Sum1 : Sum  Inputs=++++
  Out2 : Outport
  wires:
  Sum1/1 -> Out2/1
  Step/1 -> Sum1/1
  Constant/1 -> Gain/1
  From Workspace/1 -> ?
  Step1/1 -> Sum1/2
  Step2/1 -> Sum1/3
  Gain/1 -> Sum1/4

== system version4_dq/Power Plant transformer ==
  note: Network
  note: VIRTUAL RESITANCE
  Vpcc_DQ : Inport
  "VsDQ " : Inport  Port=2
  omega_ref : Inport  Port=3
  1 : Gain  Gain=inv_Lsource
  2 : Gain  Gain=Rsource
  3 : Gain  Gain=Rsource
  4 : Gain  Gain=inv_Lsource
  7 : Gain  Gain=Lsource
  Demux1 : Demux  Outputs=[vect vect]
  Demux2 : Demux  Outputs=[vect vect]
  Id : Scope
  Iline_D_int : Integrator  UpperSaturationLimit=50  LowerSaturationLimit=-1000
  Iline_Q_int : Integrator  UpperSaturationLimit=50  LowerSaturationLimit=-1000
  Iq : Scope
  Mux1 : Mux  Inputs=[vect vect]
  Mux4 : Mux  Inputs=[vect vect]
  Product1 : Product
  Product2 : Product
  Sum1 : Sum  Inputs=|+---
  Sum8 : Sum  Inputs=|+-+-
  Iline_DQ : Outport  VectorParamsAs1DForOutWhenUnconnected=off
  wires:
  7/1 -> [wL]
  [Vpcc_Q] -> Sum1/1
  [Vpcc_D] -> Sum8/1
  Demux2/1 -> Mux4/1, [Vpcc_D]
  Demux2/2 -> Mux4/2, [Vpcc_Q]
  Sum1/1 -> 4/1
  1/1 -> Iline_D_int/1
  Iline_D_int/1 -> Product1/2, Id/1, 2/1, Mux1/1
  Iline_Q_int/1 -> Mux1/2, Iq/1, Product2/2, 3/1
  Sum8/1 -> 1/1
  2/1 -> Sum8/4
  Product2/1 -> Sum8/3
  3/1 -> Sum1/4
  4/1 -> Iline_Q_int/1
  Product1/1 -> Sum1/3
  [wL] -> Product1/1, Product2/1
  Demux1/1 -> Sum8/2
  Demux1/2 -> Sum1/2
  "VsDQ "/1 -> Demux1/1
  Vpcc_DQ/1 -> Demux2/1
  Mux1/1 -> Iline_DQ/1
  omega_ref/1 -> 7/1

== system version4_dq/RC filter ==
  note: shunt capacitor
  note: Left shunt capacitor
  Iload_DQ : Inport
  "Isource_DQ " : Inport  Port=2
  omega_ref : Inport  Port=3
  1 : Gain  Commented=on  Gain=Rd
  10 : Gain  Gain=inv_Csource
  2 : Gain  Commented=on  Gain=Rd
  8 : Gain  Gain=Csource
  9 : Gain  Gain=inv_Csource
  Demux2 : Demux  Outputs=2
  Demux3 : Demux  Outputs=2
  Display1 : Display
  Display6 : Display
  Mux1 : Mux  Inputs=2
  Mux2 : Mux  Inputs=2
  Product7 : Product
  Product8 : Product
  Sum1 : Sum  Inputs=|++
  Sum14 : Sum  Inputs=|+--
  Sum15 : Sum  Inputs=|++-
  Sum2 : Sum  Inputs=|++
  Sum3 : Sum  Inputs=|+-
  Sum4 : Sum  Inputs=|+-
  Vcd : Scope
  VcpdR_int : Integrator  InitialCondition=VD0  UpperSaturationLimit=50  LowerSaturationLimit=-1000
  VcpqR_int : Integrator  InitialCondition=VQ0  UpperSaturationLimit=50  LowerSaturationLimit=-1000
  Vcq : Scope
  VpccR_DQ : Outport  VectorParamsAs1DForOutWhenUnconnected=off
  wires:
  Sum4/1 -> 2/1
  Sum3/1 -> 1/1
  Mux2/1 -> Display6/1
  2/1 -> Sum1/2
  1/1 -> Sum2/2
  Sum2/1 -> Mux1/2
  Sum1/1 -> Mux1/1
  VcpdR_int/1 -> Sum1/1, Product8/2, Vcd/1, Mux2/2
  Demux3/1 -> Sum15/3, Sum4/2
  Demux3/2 -> Sum14/2, Sum3/2
  "Isource_DQ "/1 -> Demux3/1
  Iload_DQ/1 -> Demux2/1
  Demux2/2 -> Sum14/1, Sum3/1
  Demux2/1 -> Sum15/2, Sum4/1
  9/1 -> VcpdR_int/1
  Sum14/1 -> 10/1
  [wcs] -> Product8/1, Product7/1
  VcpqR_int/1 -> Vcq/1, Product7/2, Sum2/1, Mux2/1
  Product7/1 -> Sum15/1
  10/1 -> VcpqR_int/1
  Sum15/1 -> 9/1
  Product8/1 -> Sum14/3
  Mux1/1 -> VpccR_DQ/1
  8/1 -> Display1/1, [wcs]
  omega_ref/1 -> 8/1

== system version4_dq/ROCOF test ==
  Clock : Clock
  Constant4 : Constant  Value=0
  Ramp : simulink/Sources/Ramp  slope=rocof_slope  start=Trocof_start  InitialOutput=0
  Ramp1 : simulink/Sources/Ramp  slope=rocof_slope  start=Trocof_end  InitialOutput=0
  Sample and Hold : spsSampleandHoldLib/Sample and Hold  ic=0  Ts=0
      settings: LibrarySourceBlock=|
      | sps_lib/Control/Sample and
      | Hold
  Sum : Sum  Inputs=|+-
  Switch : Switch  Criteria=u2 > Threshold  Threshold=Trocof_start  SaturateOnIntegerOverflow=off  InputSameDT=off
  Switch1 : Switch  Threshold=Trocof_end  SaturateOnIntegerOverflow=off  InputSameDT=off
  Outport : Outport
  wires:
  Clock/1 -> Switch/2, Switch1/2
  Constant4/1 -> Switch/3, Switch1/1
  Sum/1 -> Outport/1
  ? -> Switch/1
  ? -> Switch1/3
  Switch/1 -> ?
  Switch1/1 -> ?
  Ramp/1 -> Sum/1
  Ramp1/1 -> Sum/2

== system version4_dq/Subsystem ==
  V_ref_grid : Inport
  freq_ref_grid : Inport  Port=2
  angle_dist_grid : Inport  Port=3
  freq_dist_grid : Inport  Port=4
  V_dist_grid : Inport  Port=5
  Constant1 : Constant  Value=0
  Gain : Gain  Gain=2*pi
  Gain1 : Gain  Gain=1/50
  Gain2 : Gain  Gain=2*pi
  Integrator : Integrator
  Integrator1 : Integrator
  Scope : Scope  NumInputPorts=2
  Step : Step  Time=8  After=-0.1963  SampleTime=0
  Sum : Sum  Inputs=|-++
  Sum1 : Sum  Inputs=|+++
  Sum2 : Sum  Inputs=|++
  Angle : Outport
  V_mag : Outport  Port=2
  omega_ref : Outport  Port=3
  wires:
  Constant1/1 -> Gain1/1
  Gain1/1 -> Sum1/3
  Sum/1 -> Angle/1
  V_ref_grid/1 -> Sum2/1
  Sum1/1 -> Gain/1
  V_dist_grid/1 -> Sum2/2, Scope/1
  Sum2/1 -> V_mag/1, Scope/2
  freq_ref_grid/1 -> Sum1/1
  Gain/1 -> omega_ref/1, Integrator/1
  angle_dist_grid/1 -> Sum/3
  freq_dist_grid/1 -> Gain2/1, Sum1/2
  Gain2/1 -> Integrator1/1
  Integrator1/1 -> ?

== system version4_dq/WT transformer  ==
  note: Network
  note: VIRTUAL RESITANCE
  Vpcc_DQ : Inport
  "VsDQ " : Inport  Port=2
  omega_ref : Inport  Port=3
  1 : Gain  Gain=inv_Lsource
  2 : Gain  Gain=Rsource
  3 : Gain  Gain=Rsource
  4 : Gain  Gain=inv_Lsource
  7 : Gain  Gain=Lsource
  Demux1 : Demux  Outputs=2
  Demux2 : Demux  Outputs=2
  Id : Scope
  Iline_D_int : Integrator  UpperSaturationLimit=50  LowerSaturationLimit=-1000
  Iline_Q_int : Integrator  UpperSaturationLimit=50  LowerSaturationLimit=-1000
  Iq : Scope
  Mux1 : Mux  Inputs=2
  Mux4 : Mux  Inputs=2
  Product1 : Product
  Product2 : Product
  Sum1 : Sum  Inputs=|+---
  Sum8 : Sum  Inputs=|+-+-
  Iline_DQ : Outport  VectorParamsAs1DForOutWhenUnconnected=off
  wires:
  7/1 -> [wL]
  [Vpcc_Q] -> Sum1/1
  [Vpcc_D] -> Sum8/1
  Demux2/1 -> Mux4/1, [Vpcc_D]
  Demux2/2 -> Mux4/2, [Vpcc_Q]
  Sum1/1 -> 4/1
  1/1 -> Iline_D_int/1
  Iline_D_int/1 -> Product1/2, Id/1, 2/1, Mux1/1
  Iline_Q_int/1 -> Mux1/2, Iq/1, Product2/2, 3/1
  Sum8/1 -> 1/1
  2/1 -> Sum8/4
  Product2/1 -> Sum8/3
  3/1 -> Sum1/4
  4/1 -> Iline_Q_int/1
  Product1/1 -> Sum1/3
  [wL] -> Product1/1, Product2/1
  Demux1/1 -> Sum8/2
  Demux1/2 -> Sum1/2
  "VsDQ "/1 -> Demux1/1
  Vpcc_DQ/1 -> Demux2/1
  Mux1/1 -> Iline_DQ/1
  omega_ref/1 -> 7/1

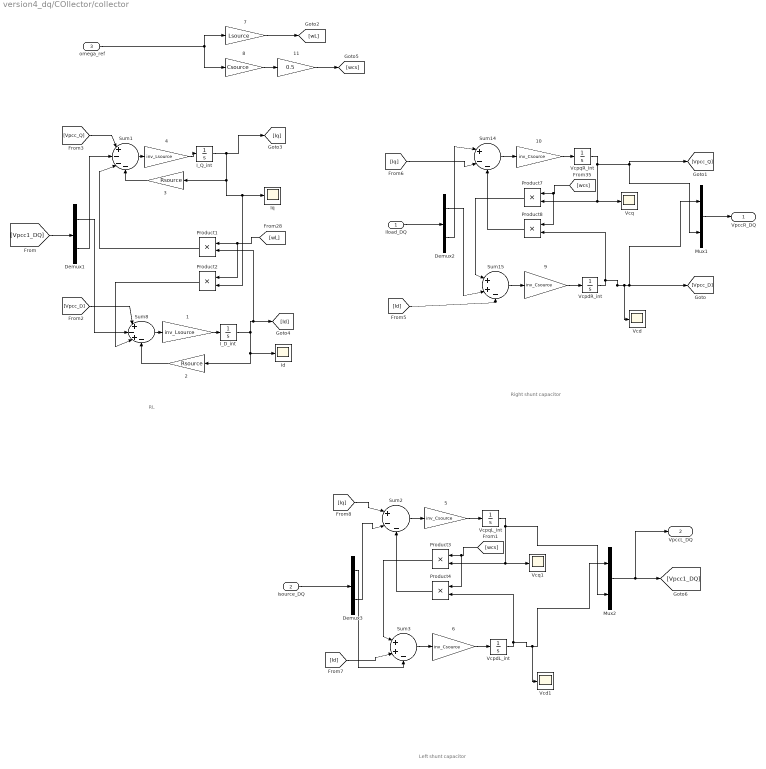
== system version4_dq/COllector/collector ==
  note: RL
  note: Right shunt capacitor
  note: Left shunt capacitor
  Iload_DQ : Inport
  "Isource_DQ " : Inport  Port=2
  omega_ref : Inport  Port=3
  1 : Gain  Gain=inv_Lsource
  {5..6,9..10} (4 alike) : Gain  Gain=inv_Csource
  11 : Gain  Gain=0.5
  2 : Gain  Gain=Rsource
  3 : Gain  Gain=Rsource
  4 : Gain  Gain=inv_Lsource
  7 : Gain  Gain=Lsource
  8 : Gain  Gain=Csource
  Demux1 : Demux  Outputs=2
  Demux2 : Demux  Outputs=2
  Demux3 : Demux  Outputs=2
  I_D_int : Integrator  UpperSaturationLimit=50  LowerSaturationLimit=-1000
  I_Q_int : Integrator  UpperSaturationLimit=50  LowerSaturationLimit=-1000
  Id : Scope
  Iq : Scope
  Mux1 : Mux  Inputs=2
  Mux2 : Mux  Inputs=2
  Product{1..4,7..8} (6 alike) : Product
  Sum1 : Sum  Inputs=|+---
  Sum14 : Sum  Inputs=|+--
  Sum15 : Sum  Inputs=|++-
  Sum2 : Sum  Inputs=|+--
  Sum3 : Sum  Inputs=|++-
  Sum8 : Sum  Inputs=|+-+-
  Vcd : Scope
  Vcd1 : Scope
  VcpdL_int : Integrator  UpperSaturationLimit=50  LowerSaturationLimit=-1000
  VcpdR_int : Integrator  UpperSaturationLimit=50  LowerSaturationLimit=-1000
  VcpqL_int : Integrator  UpperSaturationLimit=50  LowerSaturationLimit=-1000
  VcpqR_int : Integrator  UpperSaturationLimit=50  LowerSaturationLimit=-1000
  Vcq : Scope
  Vcq1 : Scope
  VpccR_DQ : Outport  VectorParamsAs1DForOutWhenUnconnected=off
  VpccL_DQ : Outport  Port=2  VectorParamsAs1DForOutWhenUnconnected=off
  wires:
  Iload_DQ/1 -> Demux2/1
  Demux2/2 -> Sum14/1
  Demux2/1 -> Sum15/2
  [wL] -> Product2/1, Product1/1
  Product1/1 -> Sum1/3
  4/1 -> I_Q_int/1
  3/1 -> Sum1/4
  Product2/1 -> Sum8/3
  2/1 -> Sum8/4
  Sum8/1 -> 1/1
  I_Q_int/1 -> 3/1, Product2/2, Iq/1, [Iq]
  I_D_int/1 -> 2/1, Id/1, Product1/2, [Id]
  1/1 -> I_D_int/1
  Sum1/1 -> 4/1
  [Vpcc_D] -> Sum8/1
  [Vpcc_Q] -> Sum1/1
  omega_ref/1 -> 8/1, 7/1
  7/1 -> [wL]
  9/1 -> VcpdR_int/1
  Sum14/1 -> 10/1
  [wcs] -> Product8/1, Product7/1
  [Id] -> Sum15/3
  VcpqR_int/1 -> Mux1/2, [Vpcc_Q], Product7/2, Vcq/1
  Product7/1 -> Sum15/1
  [Iq] -> Sum14/2
  10/1 -> VcpqR_int/1
  Sum15/1 -> 9/1
  Product8/1 -> Sum14/3
  8/1 -> 11/1
  VcpdR_int/1 -> Product8/2, Mux1/1, [Vpcc_D], Vcd/1
  Mux1/1 -> VpccR_DQ/1
  Demux1/1 -> Sum8/2
  Demux1/2 -> Sum1/2
  [Vpcc1_DQ] -> Demux1/1
  VcpdL_int/1 -> Vcd1/1, Mux2/1, Product4/2
  Product4/1 -> Sum2/3
  Sum3/1 -> 6/1
  5/1 -> VcpqL_int/1
  Demux3/2 -> Sum2/2
  Product3/1 -> Sum3/1
  VcpqL_int/1 -> Vcq1/1, Product3/2, Mux2/2
  [wcs] -> Product3/1, Product4/1
  Sum2/1 -> 5/1
  6/1 -> VcpdL_int/1
  "Isource_DQ "/1 -> Demux3/1
  Demux3/1 -> Sum3/3
  [Id] -> Sum3/2
  [Iq] -> Sum2/1
  Mux2/1 -> VpccL_DQ/1, [Vpcc1_DQ]
  11/1 -> [wcs]

== system version4_dq/GFM+WT/Current Limit Logic1 ==
  note: Circular Current limiter
  I_ref_unsat : Inport
  Abs1 : Abs
  Constant3 : Constant
  Constant4 : Constant  Value=1.2
  Demux6 : Demux  Outputs=2
  Demux7 : Demux  Outputs=[vect vect]
  Display3 : Display
  Divide : Product  Inputs=*/
  Divide1 : Product  Inputs=*/
  First-Order Filter1 : spsFirstOrderFilterLib/First-Order Filter  FilterType=Lowpass  Tc=0.002  Ts=0  Initialize=on  Vac_Init=[0, 0, 50]  Vdc_Init=0  PlotResponse=off  FreqRange="[0,  200,  1]"
  GreaterThan1 : RelationalOperator  Operator=>  OutDataTypeStr=boolean  RndMeth=Simplest  InputSameDT=off
  I_d_error2 : Scope  Commented=on
  I_d_error3 : Scope
  I_d_error5 : Scope  Commented=on
  Kip12 : Gain
  Kip13 : Gain  Gain=1/1.2
  Mux6 : Mux  Inputs=[vect vect]
  Real-Imag to Complex1 : RealImagToComplex
  Switch1 : Switch  Threshold=1  SaturateOnIntegerOverflow=off  InputSameDT=off
  Unit Delay2 : UnitDelay  InitialCondition=1  SampleTime=Ts_power  HasFrameUpgradeWarning=on
  Vmd2 : Display
  I_ref_sat : Outport
  wires:
  Mux6/1 -> I_ref_sat/1
  Divide1/1 -> Mux6/2
  Demux6/2 -> Real-Imag to Complex1/2
  Abs1/1 -> Kip13/1, I_d_error2/1, GreaterThan1/1
  Unit Delay2/1 -> Divide1/2, Divide/2
  Real-Imag to Complex1/1 -> Abs1/1
  Demux7/2 -> Divide1/1
  GreaterThan1/1 -> Switch1/2
  Demux6/1 -> Real-Imag to Complex1/1
  I_ref_unsat/1 -> Demux7/1, I_d_error5/1, Vmd2/1, First-Order Filter1/1
  Demux7/1 -> Divide/1
  Constant3/1 -> Switch1/3
  Kip13/1 -> Switch1/1
  Constant4/1 -> GreaterThan1/2
  Switch1/1 -> Kip12/1, I_d_error3/1
  Divide/1 -> Mux6/1
  Kip12/1 -> Display3/1, Unit Delay2/1
  First-Order Filter1/1 -> Demux6/1
